simulink model "abslut50_fixpt16"  (R2021b)
settings: Solver=VariableStepAuto  StartTime=0.0  StopTime=99  RelTol=1e-3
undefined symbols (not defined in the file): figd2104, xcu250
libraries: hdlBasic x391, vmcUtilities x1
(part 1 of 4)
settings Model: Creator=shu_abe  LastModifiedBy=shu_abe

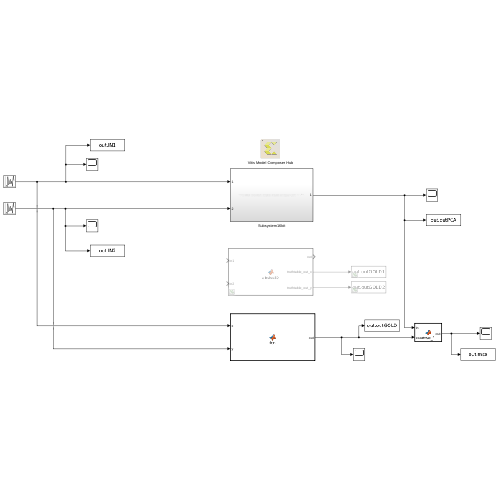
[thumbnail: Simulink's stored preview of the top-level diagram]
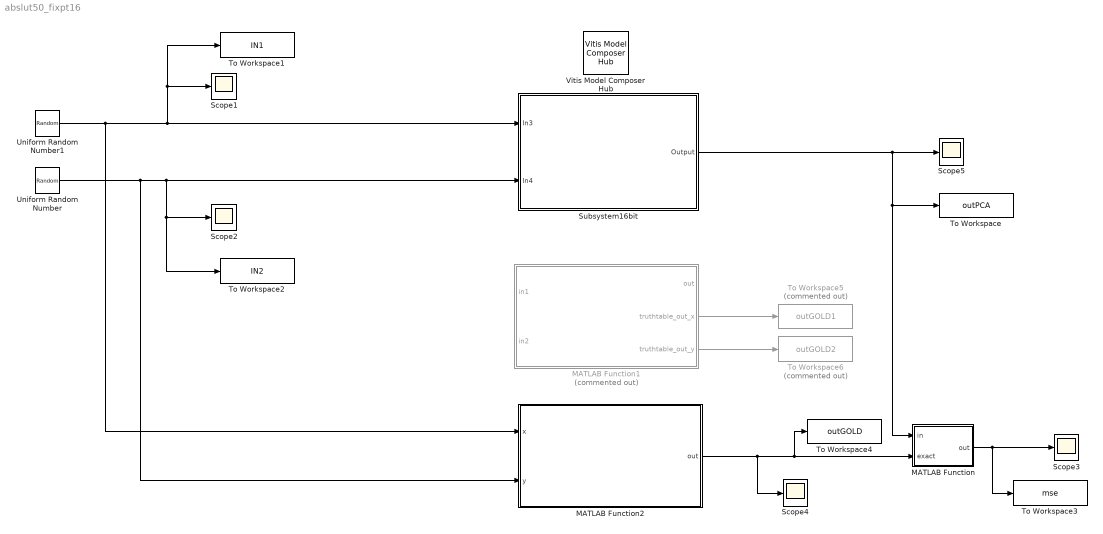
== system abslut50_fixpt16 ==
  MATLAB Function : MATLAB Function  TreatAsAtomicUnit=on
  MATLAB Function1 : MATLAB Function  Commented=on  TreatAsAtomicUnit=on
  MATLAB Function2 : MATLAB Function  TreatAsAtomicUnit=on
  Scope{1..5} (5 alike) : Scope
  Subsystem16bit : Subsystem
  To Workspace : ToWorkspace  VariableName=outPCA  SaveFormat=Structure With Time  SampleTime=1
  To Workspace1 : ToWorkspace  VariableName=IN1  SaveFormat=Structure With Time  SampleTime=-1
  To Workspace2 : ToWorkspace  VariableName=IN2  SaveFormat=Structure With Time  SampleTime=-1
  To Workspace3 : ToWorkspace  VariableName=mse  SaveFormat=Structure With Time  SampleTime=1
  To Workspace4 : ToWorkspace  VariableName=outGOLD  SaveFormat=Structure With Time  SampleTime=1
  To Workspace5 : ToWorkspace  Commented=on  VariableName=outGOLD1  SaveFormat=Structure With Time  SampleTime=1
  To Workspace6 : ToWorkspace  Commented=on  VariableName=outGOLD2  SaveFormat=Structure With Time  SampleTime=1
  Uniform Random Number : UniformRandomNumber  SampleTime=1
  Uniform Random Number1 : UniformRandomNumber  Seed=1  SampleTime=1
  Vitis Model Composer Hub : vmcUtilities/Vitis Model Composer Hub  Tag=genX  CodeGeneration=off  SubsystemName=<enter or select subsystem name>  TargetDirectory=./code  ExportType=HLS C++ code  IpVendor=xilinx.com  IpLibrary=hls  IpVersion=1.0  IpHWLanguage=Verilog  AieCompilerOptions={}  CreateTestbench=off  TestbenchStackSize=10  RunAieSim=off  AieSimTimeout=50000  RunAieSimProfiling=off  LaunchVitisAnalyzer=off  PlotOutput=off  RunX86Sim=off  X86SimTimeout=10  GenHwImage=off  PlatformType=Not Specified  HwSystemType=Baremetal  HwValidationTarget=hw  ProjDevice=Alveo U250 Data Center Accelerator Card (xcu250-figd2104-2L-e)  ProjDevicePart=xcu250-figd2104-2L-e  SamplePeriod=-1  ClockFrequency=200  DataPathParallelism=1  xilinxfamily=virtexuplus  part=xcu250  speed=-2L-e  package=figd2104  directory=./abs19  testbench=on  incr_netlist=off  synthesis_tool=Vivado  clock_wrapper=Clock Enables  dbl_ovrd=According to Block Masks  dcm_input_clock_period=10  sysclk_period=100  simulink_period=1  eval_field=0
  wires:
  MATLAB Function/1(out) -> Scope3/1, To Workspace3/1
  Subsystem16bit/1(Output) -> Scope5/1, MATLAB Function/1(in), To Workspace/1
  MATLAB Function2/1(out) -> Scope4/1, To Workspace4/1, MATLAB Function/2(exact)
  Uniform Random Number1/1 -> MATLAB Function2/1(x), To Workspace1/1, Scope1/1, Subsystem16bit/1(In3)
  Uniform Random Number/1 -> MATLAB Function2/2(y), Subsystem16bit/2(In4), To Workspace2/1, Scope2/1
  MATLAB Function1/2(truthtable_out_x) -> To Workspace5/1
  MATLAB Function1/3(truthtable_out_y) -> To Workspace6/1
